simulink model "mpc3"  (R2018b)
settings: Solver=VariableStepAuto  StartTime=0.0  StopTime=10.0  RelTol=1e-3
values from neighbouring files (symbols this model uses):
  A1 = [0 0 1 0 ; 0 0 0 1 ; 0 A132 A133 A134 ; 0 A142 A143 A144]    [NXTway_model.m]
  B1 = [0 0 ; 0 0 ; B13 B13 ; B14 B14]    [NXTway_model.m]
undefined symbols (not defined in the file or in its folder): Continuous, Time
libraries: simulink x1, ctrlSharedLib x1, mpclib x1
settings Model: Creator=jimve  LastModifiedBy=jimve

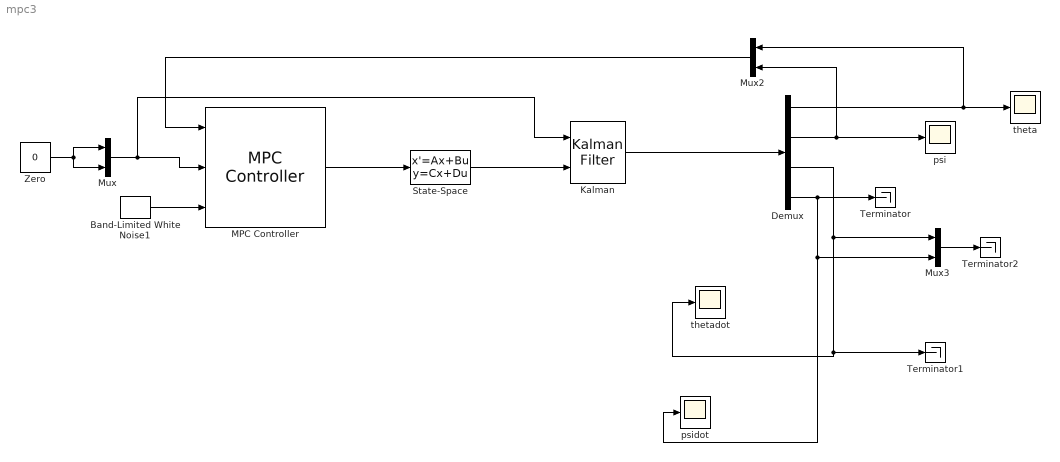
== system mpc3 ==
  Band-Limited White Noise1 : simulink/Sources/Band-Limited White Noise  Cov=[0.01]  Ts=0.1  seed=[23341]
  Demux : Demux
  Kalman : ctrlSharedLib/Kalman Filter  TimeDomain=Continuous-Time  UseCurrentEstimator=on  ModelSource=LTI State-Space Variable  ModelSourceVariable=sys1  A=0.95  B=1  C=1  D=0  NumberOfStates=1  NumberOfInputs=1  NumberOfOutputs=1  InitialEstimateSource=Dialog  X0=[0 -0.2 0 0]  P0=10  UseK=off  UseGH=off  NumberOfProcessNoiseInputs=1  G=1  TimeInvariantG=on  H=0  TimeInvariantH=on  Q=0.05  TimeInvariantQ=on  R=1  TimeInvariantR=on  N=0  TimeInvariantN=on  AddInputPort=on  AddEnablePort=off  OutputEstimatedY=off  OutputP=off  Ts=-1
      settings: SourceProductBaseCode=CT
  MPC Controller : mpclib/MPC Controller  SCDEnableBlockLinearizationSpecification=on  mpcobj=mpc1  is_multiple=0  enable_value=0  return_u0=off  updateMPCinCallerWorkspace=on  md_inport=on  mv_inport=off  return_cost=off  return_mvseq=off  return_qpstatus=off  return_xseq=off  return_state=off  return_ovseq=off  state_inport=off  umin_inport=off  umax_inport=off  ymin_inport=off  ymax_inport=off  cc_inport=off  ywt_inport=off  uwt_inport=off  duwt_inport=off  rhoeps_inport=off  uref_inport=off  n_ts=0.1  n_p=10  n_mv=2  n_md=1  n_ud=0  n_mo=2  n_uo=0  BlockDataType=double  SampleTimeInherited=off  switch_inport=off
  Mux : Mux  Inputs=2
  Mux2 : Mux  Inputs=2
  Mux3 : Mux  Inputs=2
  State-Space : StateSpace  A=A1  B=B1  C=[1 0 0 0 ; 0 0 0 1]  D=zeros(2,2)  InitialCondition=[0 -0.2 0 0]
  Terminator : Terminator
  Terminator1 : Terminator
  Terminator2 : Terminator
  Zero : Constant  Value=0  OutDataTypeStr=Inherit: Inherit via back propagation
  psi : Scope
  psidot : Scope
  theta : Scope
  "thetadot " : Scope
  wires:
  Zero/1 -> Mux/2, Mux/1
  State-Space/1 -> Kalman/2
  Band-Limited White Noise1/1 -> MPC Controller/3
  Demux/4 -> Mux3/2, psidot/1, Terminator/1
  Kalman/1 -> Demux/1
  Demux/3 -> Mux3/1, "thetadot "/1, Terminator1/1
  MPC Controller/1 -> State-Space/1
  Mux2/1 -> MPC Controller/1
  Mux3/1 -> Terminator2/1
  Demux/1 -> Mux2/1, theta/1
  Demux/2 -> Mux2/2, psi/1
  Mux/1 -> Kalman/1, MPC Controller/2
